simulink model "OrbiterPhysicalSystem"  (R2022b)
settings: Solver=VariableStepAuto  StartTime=0.0  StopTime=100  RelTol=1e-3
libraries: fl_lib x62, nesl_utility x10
settings Model: Creator=aless  LastModifiedBy=aless

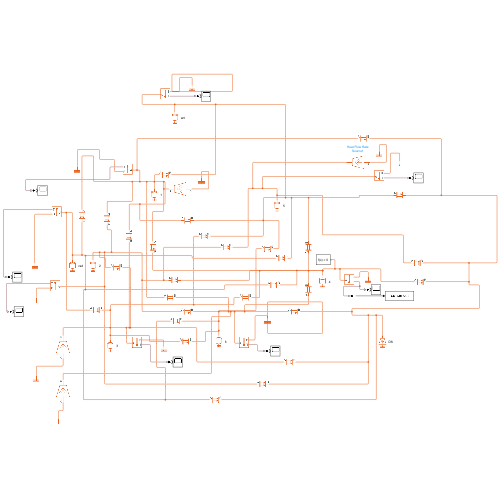
[thumbnail: Simulink's stored preview of the top-level diagram]
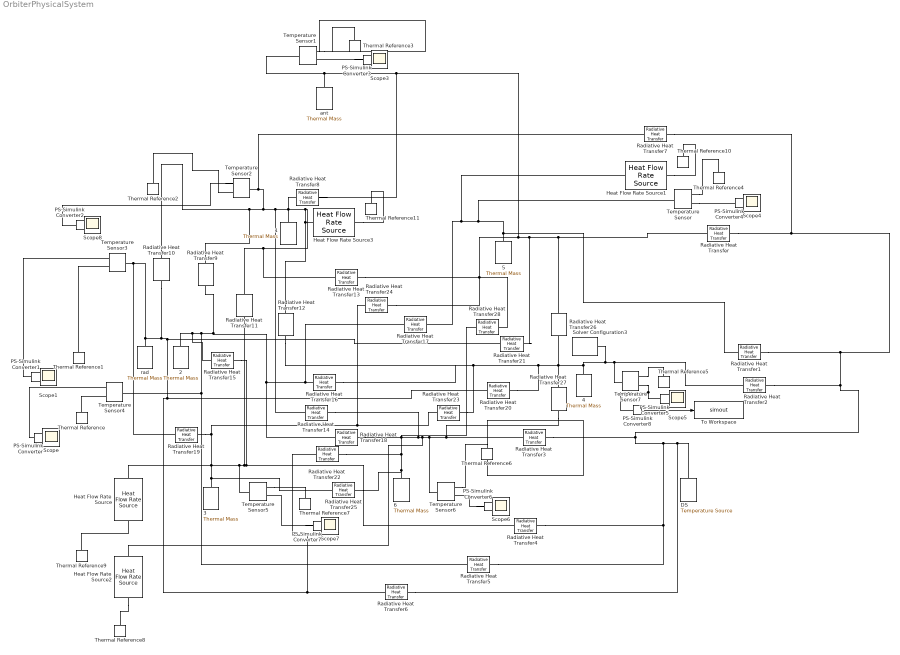
== system OrbiterPhysicalSystem ==
  {1..6} (6 alike) : fl_lib/Thermal/Thermal Elements/Thermal Mass  mass=1 kg  sp_heat=447 J/(K*kg)  num_ports=foundation.enum.numPorts2.one  T_specify=off  T_priority=High  T=300 K  T_nominal_specify=on  T_nominal_unit=K  T_nominal_value=T0  Q_specify=off  Q_priority=None  Q=0 W  Q_nominal_specify=off  Q_nominal_unit=W  Q_nominal_value=1
  DS : fl_lib/Thermal/Thermal Sources/Temperature Source  temperature=4 K
  Heat Flow Rate Source : fl_lib/Thermal/Thermal Sources/Heat Flow Rate Source  heat_flow=Q_ext_hot3 W
      settings: InternalSimscapePortConfiguration="{\"Bottom\":[],\"Left\":[{\"id\":\"B\",\"label\":\"B\",\"type\":\"foundation.thermal.thermal\"}],\"Right\":[{\"id\":\"A\",\"label\":\"A\",\"type\":\"foundation.thermal.thermal\"}],\"Top\":[]}"
  Heat Flow Rate Source1 : fl_lib/Thermal/Thermal Sources/Heat Flow Rate Source  heat_flow=Q_ext_hot5 W
      settings: InternalSimscapePortConfiguration="{\"Bottom\":[],\"Left\":[{\"id\":\"B\",\"label\":\"B\",\"type\":\"foundation.thermal.thermal\"}],\"Right\":[{\"id\":\"A\",\"label\":\"A\",\"type\":\"foundation.thermal.thermal\"}],\"Top\":[]}"
  Heat Flow Rate Source2 : fl_lib/Thermal/Thermal Sources/Heat Flow Rate Source  heat_flow=Q_ext_hot3 W
      settings: InternalSimscapePortConfiguration="{\"Bottom\":[],\"Left\":[{\"id\":\"B\",\"label\":\"B\",\"type\":\"foundation.thermal.thermal\"}],\"Right\":[{\"id\":\"A\",\"label\":\"A\",\"type\":\"foundation.thermal.thermal\"}],\"Top\":[]}"
  Heat Flow Rate Source3 : fl_lib/Thermal/Thermal Sources/Heat Flow Rate Source  heat_flow=Q_hot W
      settings: InternalSimscapePortConfiguration="{\"Bottom\":[],\"Left\":[{\"id\":\"B\",\"label\":\"B\",\"type\":\"foundation.thermal.thermal\"}],\"Right\":[{\"id\":\"A\",\"label\":\"A\",\"type\":\"foundation.thermal.thermal\"}],\"Top\":[]}"
  PS-Simulink Converter{,1..8} (9 alike) : nesl_utility/PS-Simulink Converter  PhysicalDomain=network_engine_domain  SubClassName=ps_output  LeftPortType=input  RightPortType=output  PseudoPeriodic=off  Frequencies=[]  VectorFormat=inherit  Unit=inherit  AffineConversion=off
  Radiative Heat Transfer : fl_lib/Thermal/Thermal Elements/Radiative Heat Transfer  area=A_ant m^2  rad_tr_coeff=R.R_ant0 W/(K^4*m^2)  T_specify=off  T_priority=None  T=0 K  T_nominal_specify=off  T_nominal_unit=K  T_nominal_value=1  Q_specify=off  Q_priority=None  Q=0 W  Q_nominal_specify=off  Q_nominal_unit=W  Q_nominal_value=1
      settings: InternalSimscapePortConfiguration="{\"Bottom\":[],\"Left\":[{\"id\":\"A\",\"label\":\"A\",\"type\":\"foundation.thermal.thermal\"}],\"Right\":[{\"id\":\"B\",\"label\":\"B\",\"type\":\"foundation.thermal.thermal\"}],\"Top\":[]}"
  Radiative Heat Transfer1 : fl_lib/Thermal/Thermal Elements/Radiative Heat Transfer  area=A5 m^2  rad_tr_coeff=R.R_50 W/(K^4*m^2)  T_specify=off  T_priority=None  T=0 K  T_nominal_specify=off  T_nominal_unit=K  T_nominal_value=1  Q_specify=off  Q_priority=None  Q=0 W  Q_nominal_specify=off  Q_nominal_unit=W  Q_nominal_value=1
      settings: InternalSimscapePortConfiguration="{\"Bottom\":[],\"Left\":[{\"id\":\"A\",\"label\":\"A\",\"type\":\"foundation.thermal.thermal\"}],\"Right\":[{\"id\":\"B\",\"label\":\"B\",\"type\":\"foundation.thermal.thermal\"}],\"Top\":[]}"
  Radiative Heat Transfer10 : fl_lib/Thermal/Thermal Elements/Radiative Heat Transfer  area=A1 m^2  rad_tr_coeff=R.R_1rad W/(K^4*m^2)  T_specify=off  T_priority=None  T=0 K  T_nominal_specify=off  T_nominal_unit=K  T_nominal_value=1  Q_specify=off  Q_priority=None  Q=0 W  Q_nominal_specify=off  Q_nominal_unit=W  Q_nominal_value=1
      settings: InternalSimscapePortConfiguration="{\"Bottom\":[],\"Left\":[{\"id\":\"A\",\"label\":\"A\",\"type\":\"foundation.thermal.thermal\"}],\"Right\":[{\"id\":\"B\",\"label\":\"B\",\"type\":\"foundation.thermal.thermal\"}],\"Top\":[]}"
  Radiative Heat Transfer11 : fl_lib/Thermal/Thermal Elements/Radiative Heat Transfer  area=A1 m^2  rad_tr_coeff=R.R_13 W/(K^4*m^2)  T_specify=off  T_priority=None  T=0 K  T_nominal_specify=off  T_nominal_unit=K  T_nominal_value=1  Q_specify=off  Q_priority=None  Q=0 W  Q_nominal_specify=off  Q_nominal_unit=W  Q_nominal_value=1
      settings: InternalSimscapePortConfiguration="{\"Bottom\":[],\"Left\":[{\"id\":\"A\",\"label\":\"A\",\"type\":\"foundation.thermal.thermal\"}],\"Right\":[{\"id\":\"B\",\"label\":\"B\",\"type\":\"foundation.thermal.thermal\"}],\"Top\":[]}"
  Radiative Heat Transfer12 : fl_lib/Thermal/Thermal Elements/Radiative Heat Transfer  area=A1 m^2  rad_tr_coeff=R.R_14 W/(K^4*m^2)  T_specify=off  T_priority=None  T=0 K  T_nominal_specify=off  T_nominal_unit=K  T_nominal_value=1  Q_specify=off  Q_priority=None  Q=0 W  Q_nominal_specify=off  Q_nominal_unit=W  Q_nominal_value=1
      settings: InternalSimscapePortConfiguration="{\"Bottom\":[],\"Left\":[{\"id\":\"A\",\"label\":\"A\",\"type\":\"foundation.thermal.thermal\"}],\"Right\":[{\"id\":\"B\",\"label\":\"B\",\"type\":\"foundation.thermal.thermal\"}],\"Top\":[]}"
  Radiative Heat Transfer13 : fl_lib/Thermal/Thermal Elements/Radiative Heat Transfer  area=A1 m^2  rad_tr_coeff=R.R_15 W/(K^4*m^2)  T_specify=off  T_priority=None  T=0 K  T_nominal_specify=off  T_nominal_unit=K  T_nominal_value=1  Q_specify=off  Q_priority=None  Q=0 W  Q_nominal_specify=off  Q_nominal_unit=W  Q_nominal_value=1
      settings: InternalSimscapePortConfiguration="{\"Bottom\":[],\"Left\":[{\"id\":\"A\",\"label\":\"A\",\"type\":\"foundation.thermal.thermal\"}],\"Right\":[{\"id\":\"B\",\"label\":\"B\",\"type\":\"foundation.thermal.thermal\"}],\"Top\":[]}"
  Radiative Heat Transfer14 : fl_lib/Thermal/Thermal Elements/Radiative Heat Transfer  area=A1 m^2  rad_tr_coeff=R.R_16 W/(K^4*m^2)  T_specify=off  T_priority=None  T=0 K  T_nominal_specify=off  T_nominal_unit=K  T_nominal_value=1  Q_specify=off  Q_priority=None  Q=0 W  Q_nominal_specify=off  Q_nominal_unit=W  Q_nominal_value=1
      settings: InternalSimscapePortConfiguration="{\"Bottom\":[],\"Left\":[{\"id\":\"A\",\"label\":\"A\",\"type\":\"foundation.thermal.thermal\"}],\"Right\":[{\"id\":\"B\",\"label\":\"B\",\"type\":\"foundation.thermal.thermal\"}],\"Top\":[]}"
  Radiative Heat Transfer15 : fl_lib/Thermal/Thermal Elements/Radiative Heat Transfer  area=A2 m^2  rad_tr_coeff=R.R_23 W/(K^4*m^2)  T_specify=off  T_priority=None  T=0 K  T_nominal_specify=off  T_nominal_unit=K  T_nominal_value=1  Q_specify=off  Q_priority=None  Q=0 W  Q_nominal_specify=off  Q_nominal_unit=W  Q_nominal_value=1
      settings: InternalSimscapePortConfiguration="{\"Bottom\":[],\"Left\":[{\"id\":\"A\",\"label\":\"A\",\"type\":\"foundation.thermal.thermal\"}],\"Right\":[{\"id\":\"B\",\"label\":\"B\",\"type\":\"foundation.thermal.thermal\"}],\"Top\":[]}"
  Radiative Heat Transfer16 : fl_lib/Thermal/Thermal Elements/Radiative Heat Transfer  area=A2 m^2  rad_tr_coeff=R.R_24 W/(K^4*m^2)  T_specify=off  T_priority=None  T=0 K  T_nominal_specify=off  T_nominal_unit=K  T_nominal_value=1  Q_specify=off  Q_priority=None  Q=0 W  Q_nominal_specify=off  Q_nominal_unit=W  Q_nominal_value=1
      settings: InternalSimscapePortConfiguration="{\"Bottom\":[],\"Left\":[{\"id\":\"A\",\"label\":\"A\",\"type\":\"foundation.thermal.thermal\"}],\"Right\":[{\"id\":\"B\",\"label\":\"B\",\"type\":\"foundation.thermal.thermal\"}],\"Top\":[]}"
  Radiative Heat Transfer17 : fl_lib/Thermal/Thermal Elements/Radiative Heat Transfer  area=A2 m^2  rad_tr_coeff=R.R_25 W/(K^4*m^2)  T_specify=off  T_priority=None  T=0 K  T_nominal_specify=off  T_nominal_unit=K  T_nominal_value=1  Q_specify=off  Q_priority=None  Q=0 W  Q_nominal_specify=off  Q_nominal_unit=W  Q_nominal_value=1
      settings: InternalSimscapePortConfiguration="{\"Bottom\":[],\"Left\":[{\"id\":\"A\",\"label\":\"A\",\"type\":\"foundation.thermal.thermal\"}],\"Right\":[{\"id\":\"B\",\"label\":\"B\",\"type\":\"foundation.thermal.thermal\"}],\"Top\":[]}"
  Radiative Heat Transfer18 : fl_lib/Thermal/Thermal Elements/Radiative Heat Transfer  area=A2 m^2  rad_tr_coeff=R.R_26 W/(K^4*m^2)  T_specify=off  T_priority=None  T=0 K  T_nominal_specify=off  T_nominal_unit=K  T_nominal_value=1  Q_specify=off  Q_priority=None  Q=0 W  Q_nominal_specify=off  Q_nominal_unit=W  Q_nominal_value=1
      settings: InternalSimscapePortConfiguration="{\"Bottom\":[],\"Left\":[{\"id\":\"A\",\"label\":\"A\",\"type\":\"foundation.thermal.thermal\"}],\"Right\":[{\"id\":\"B\",\"label\":\"B\",\"type\":\"foundation.thermal.thermal\"}],\"Top\":[]}"
  Radiative Heat Transfer19 : fl_lib/Thermal/Thermal Elements/Radiative Heat Transfer  area=A_rad_tot m^2  rad_tr_coeff=R.R_rad3 W/(K^4*m^2)  T_specify=off  T_priority=None  T=0 K  T_nominal_specify=off  T_nominal_unit=K  T_nominal_value=1  Q_specify=off  Q_priority=None  Q=0 W  Q_nominal_specify=off  Q_nominal_unit=W  Q_nominal_value=1
      settings: InternalSimscapePortConfiguration="{\"Bottom\":[],\"Left\":[{\"id\":\"A\",\"label\":\"A\",\"type\":\"foundation.thermal.thermal\"}],\"Right\":[{\"id\":\"B\",\"label\":\"B\",\"type\":\"foundation.thermal.thermal\"}],\"Top\":[]}"
  Radiative Heat Transfer2 : fl_lib/Thermal/Thermal Elements/Radiative Heat Transfer  area=A4 m^2  rad_tr_coeff=R.R_40 W/(K^4*m^2)  T_specify=off  T_priority=None  T=0 K  T_nominal_specify=off  T_nominal_unit=K  T_nominal_value=1  Q_specify=off  Q_priority=None  Q=0 W  Q_nominal_specify=off  Q_nominal_unit=W  Q_nominal_value=1
      settings: InternalSimscapePortConfiguration="{\"Bottom\":[],\"Left\":[{\"id\":\"A\",\"label\":\"A\",\"type\":\"foundation.thermal.thermal\"}],\"Right\":[{\"id\":\"B\",\"label\":\"B\",\"type\":\"foundation.thermal.thermal\"}],\"Top\":[]}"
  Radiative Heat Transfer20 : fl_lib/Thermal/Thermal Elements/Radiative Heat Transfer  area=A_rad_tot m^2  rad_tr_coeff=R.R_rad4 W/(K^4*m^2)  T_specify=off  T_priority=None  T=0 K  T_nominal_specify=off  T_nominal_unit=K  T_nominal_value=1  Q_specify=off  Q_priority=None  Q=0 W  Q_nominal_specify=off  Q_nominal_unit=W  Q_nominal_value=1
      settings: InternalSimscapePortConfiguration="{\"Bottom\":[],\"Left\":[{\"id\":\"A\",\"label\":\"A\",\"type\":\"foundation.thermal.thermal\"}],\"Right\":[{\"id\":\"B\",\"label\":\"B\",\"type\":\"foundation.thermal.thermal\"}],\"Top\":[]}"
  Radiative Heat Transfer21 : fl_lib/Thermal/Thermal Elements/Radiative Heat Transfer  area=A_rad_tot m^2  rad_tr_coeff=R.R_rad5 W/(K^4*m^2)  T_specify=off  T_priority=None  T=0 K  T_nominal_specify=off  T_nominal_unit=K  T_nominal_value=1  Q_specify=off  Q_priority=None  Q=0 W  Q_nominal_specify=off  Q_nominal_unit=W  Q_nominal_value=1
      settings: InternalSimscapePortConfiguration="{\"Bottom\":[],\"Left\":[{\"id\":\"A\",\"label\":\"A\",\"type\":\"foundation.thermal.thermal\"}],\"Right\":[{\"id\":\"B\",\"label\":\"B\",\"type\":\"foundation.thermal.thermal\"}],\"Top\":[]}"
  Radiative Heat Transfer22 : fl_lib/Thermal/Thermal Elements/Radiative Heat Transfer  area=A_rad_tot m^2  rad_tr_coeff=R.R_rad6 W/(K^4*m^2)  T_specify=off  T_priority=None  T=0 K  T_nominal_specify=off  T_nominal_unit=K  T_nominal_value=1  Q_specify=off  Q_priority=None  Q=0 W  Q_nominal_specify=off  Q_nominal_unit=W  Q_nominal_value=1
      settings: InternalSimscapePortConfiguration="{\"Bottom\":[],\"Left\":[{\"id\":\"A\",\"label\":\"A\",\"type\":\"foundation.thermal.thermal\"}],\"Right\":[{\"id\":\"B\",\"label\":\"B\",\"type\":\"foundation.thermal.thermal\"}],\"Top\":[]}"
  Radiative Heat Transfer23 : fl_lib/Thermal/Thermal Elements/Radiative Heat Transfer  area=A3 m^2  rad_tr_coeff=R.R_34 W/(K^4*m^2)  T_specify=off  T_priority=None  T=0 K  T_nominal_specify=off  T_nominal_unit=K  T_nominal_value=1  Q_specify=off  Q_priority=None  Q=0 W  Q_nominal_specify=off  Q_nominal_unit=W  Q_nominal_value=1
      settings: InternalSimscapePortConfiguration="{\"Bottom\":[],\"Left\":[{\"id\":\"A\",\"label\":\"A\",\"type\":\"foundation.thermal.thermal\"}],\"Right\":[{\"id\":\"B\",\"label\":\"B\",\"type\":\"foundation.thermal.thermal\"}],\"Top\":[]}"
  Radiative Heat Transfer24 : fl_lib/Thermal/Thermal Elements/Radiative Heat Transfer  area=A3 m^2  rad_tr_coeff=R.R_35 W/(K^4*m^2)  T_specify=off  T_priority=None  T=0 K  T_nominal_specify=off  T_nominal_unit=K  T_nominal_value=1  Q_specify=off  Q_priority=None  Q=0 W  Q_nominal_specify=off  Q_nominal_unit=W  Q_nominal_value=1
      settings: InternalSimscapePortConfiguration="{\"Bottom\":[],\"Left\":[{\"id\":\"A\",\"label\":\"A\",\"type\":\"foundation.thermal.thermal\"}],\"Right\":[{\"id\":\"B\",\"label\":\"B\",\"type\":\"foundation.thermal.thermal\"}],\"Top\":[]}"
  Radiative Heat Transfer25 : fl_lib/Thermal/Thermal Elements/Radiative Heat Transfer  area=A3 m^2  rad_tr_coeff=R.R_36 W/(K^4*m^2)  T_specify=off  T_priority=None  T=0 K  T_nominal_specify=off  T_nominal_unit=K  T_nominal_value=1  Q_specify=off  Q_priority=None  Q=0 W  Q_nominal_specify=off  Q_nominal_unit=W  Q_nominal_value=1
      settings: InternalSimscapePortConfiguration="{\"Bottom\":[],\"Left\":[{\"id\":\"A\",\"label\":\"A\",\"type\":\"foundation.thermal.thermal\"}],\"Right\":[{\"id\":\"B\",\"label\":\"B\",\"type\":\"foundation.thermal.thermal\"}],\"Top\":[]}"
  Radiative Heat Transfer26 : fl_lib/Thermal/Thermal Elements/Radiative Heat Transfer  area=A4 m^2  rad_tr_coeff=R.R_45 W/(K^4*m^2)  T_specify=off  T_priority=None  T=0 K  T_nominal_specify=off  T_nominal_unit=K  T_nominal_value=1  Q_specify=off  Q_priority=None  Q=0 W  Q_nominal_specify=off  Q_nominal_unit=W  Q_nominal_value=1
      settings: InternalSimscapePortConfiguration="{\"Bottom\":[],\"Left\":[{\"id\":\"A\",\"label\":\"A\",\"type\":\"foundation.thermal.thermal\"}],\"Right\":[{\"id\":\"B\",\"label\":\"B\",\"type\":\"foundation.thermal.thermal\"}],\"Top\":[]}"
  Radiative Heat Transfer27 : fl_lib/Thermal/Thermal Elements/Radiative Heat Transfer  area=A4 m^2  rad_tr_coeff=R.R_46 W/(K^4*m^2)  T_specify=off  T_priority=None  T=0 K  T_nominal_specify=off  T_nominal_unit=K  T_nominal_value=1  Q_specify=off  Q_priority=None  Q=0 W  Q_nominal_specify=off  Q_nominal_unit=W  Q_nominal_value=1
      settings: InternalSimscapePortConfiguration="{\"Bottom\":[],\"Left\":[{\"id\":\"A\",\"label\":\"A\",\"type\":\"foundation.thermal.thermal\"}],\"Right\":[{\"id\":\"B\",\"label\":\"B\",\"type\":\"foundation.thermal.thermal\"}],\"Top\":[]}"
  Radiative Heat Transfer28 : fl_lib/Thermal/Thermal Elements/Radiative Heat Transfer  area=A5 m^2  rad_tr_coeff=R.R_56 W/(K^4*m^2)  T_specify=off  T_priority=None  T=0 K  T_nominal_specify=off  T_nominal_unit=K  T_nominal_value=1  Q_specify=off  Q_priority=None  Q=0 W  Q_nominal_specify=off  Q_nominal_unit=W  Q_nominal_value=1
      settings: InternalSimscapePortConfiguration="{\"Bottom\":[],\"Left\":[{\"id\":\"A\",\"label\":\"A\",\"type\":\"foundation.thermal.thermal\"}],\"Right\":[{\"id\":\"B\",\"label\":\"B\",\"type\":\"foundation.thermal.thermal\"}],\"Top\":[]}"
  Radiative Heat Transfer3 : fl_lib/Thermal/Thermal Elements/Radiative Heat Transfer  area=A6 m^2  rad_tr_coeff=R.R_60 W/(K^4*m^2)  T_specify=off  T_priority=None  T=0 K  T_nominal_specify=off  T_nominal_unit=K  T_nominal_value=1  Q_specify=off  Q_priority=None  Q=0 W  Q_nominal_specify=off  Q_nominal_unit=W  Q_nominal_value=1
      settings: InternalSimscapePortConfiguration="{\"Bottom\":[],\"Left\":[{\"id\":\"A\",\"label\":\"A\",\"type\":\"foundation.thermal.thermal\"}],\"Right\":[{\"id\":\"B\",\"label\":\"B\",\"type\":\"foundation.thermal.thermal\"}],\"Top\":[]}"
  Radiative Heat Transfer4 : fl_lib/Thermal/Thermal Elements/Radiative Heat Transfer  area=A3 m^2  rad_tr_coeff=R.R_30 W/(K^4*m^2)  T_specify=off  T_priority=None  T=0 K  T_nominal_specify=off  T_nominal_unit=K  T_nominal_value=1  Q_specify=off  Q_priority=None  Q=0 W  Q_nominal_specify=off  Q_nominal_unit=W  Q_nominal_value=1
      settings: InternalSimscapePortConfiguration="{\"Bottom\":[],\"Left\":[{\"id\":\"A\",\"label\":\"A\",\"type\":\"foundation.thermal.thermal\"}],\"Right\":[{\"id\":\"B\",\"label\":\"B\",\"type\":\"foundation.thermal.thermal\"}],\"Top\":[]}"
  Radiative Heat Transfer5 : fl_lib/Thermal/Thermal Elements/Radiative Heat Transfer  area=A2 m^2  rad_tr_coeff=R.R_20 W/(K^4*m^2)  T_specify=off  T_priority=None  T=0 K  T_nominal_specify=off  T_nominal_unit=K  T_nominal_value=1  Q_specify=off  Q_priority=None  Q=0 W  Q_nominal_specify=off  Q_nominal_unit=W  Q_nominal_value=1
      settings: InternalSimscapePortConfiguration="{\"Bottom\":[],\"Left\":[{\"id\":\"A\",\"label\":\"A\",\"type\":\"foundation.thermal.thermal\"}],\"Right\":[{\"id\":\"B\",\"label\":\"B\",\"type\":\"foundation.thermal.thermal\"}],\"Top\":[]}"
  Radiative Heat Transfer6 : fl_lib/Thermal/Thermal Elements/Radiative Heat Transfer  area=A_rad_tot m^2  rad_tr_coeff=R.R_rad0 W/(K^4*m^2)  T_specify=off  T_priority=None  T=0 K  T_nominal_specify=off  T_nominal_unit=K  T_nominal_value=1  Q_specify=off  Q_priority=None  Q=0 W  Q_nominal_specify=off  Q_nominal_unit=W  Q_nominal_value=1
      settings: InternalSimscapePortConfiguration="{\"Bottom\":[],\"Left\":[{\"id\":\"A\",\"label\":\"A\",\"type\":\"foundation.thermal.thermal\"}],\"Right\":[{\"id\":\"B\",\"label\":\"B\",\"type\":\"foundation.thermal.thermal\"}],\"Top\":[]}"
  Radiative Heat Transfer7 : fl_lib/Thermal/Thermal Elements/Radiative Heat Transfer  area=A1 m^2  rad_tr_coeff=R.R_10 W/(K^4*m^2)  T_specify=off  T_priority=None  T=0 K  T_nominal_specify=off  T_nominal_unit=K  T_nominal_value=1  Q_specify=off  Q_priority=None  Q=0 W  Q_nominal_specify=off  Q_nominal_unit=W  Q_nominal_value=1
      settings: InternalSimscapePortConfiguration="{\"Bottom\":[],\"Left\":[{\"id\":\"A\",\"label\":\"A\",\"type\":\"foundation.thermal.thermal\"}],\"Right\":[{\"id\":\"B\",\"label\":\"B\",\"type\":\"foundation.thermal.thermal\"}],\"Top\":[]}"
  Radiative Heat Transfer8 : fl_lib/Thermal/Thermal Elements/Radiative Heat Transfer  area=A1 m^2  rad_tr_coeff=R.R_1ant W/(K^4*m^2)  T_specify=off  T_priority=None  T=0 K  T_nominal_specify=off  T_nominal_unit=K  T_nominal_value=1  Q_specify=off  Q_priority=None  Q=0 W  Q_nominal_specify=off  Q_nominal_unit=W  Q_nominal_value=1
      settings: InternalSimscapePortConfiguration="{\"Bottom\":[],\"Left\":[{\"id\":\"A\",\"label\":\"A\",\"type\":\"foundation.thermal.thermal\"}],\"Right\":[{\"id\":\"B\",\"label\":\"B\",\"type\":\"foundation.thermal.thermal\"}],\"Top\":[]}"
  Radiative Heat Transfer9 : fl_lib/Thermal/Thermal Elements/Radiative Heat Transfer  area=A1 m^2  rad_tr_coeff=R.R_12 W/(K^4*m^2)  T_specify=off  T_priority=None  T=0 K  T_nominal_specify=off  T_nominal_unit=K  T_nominal_value=1  Q_specify=off  Q_priority=None  Q=0 W  Q_nominal_specify=off  Q_nominal_unit=W  Q_nominal_value=1
      settings: InternalSimscapePortConfiguration="{\"Bottom\":[],\"Left\":[{\"id\":\"A\",\"label\":\"A\",\"type\":\"foundation.thermal.thermal\"}],\"Right\":[{\"id\":\"B\",\"label\":\"B\",\"type\":\"foundation.thermal.thermal\"}],\"Top\":[]}"
  Scope{,1,3..8} (8 alike) : Scope
  Solver Configuration3 : nesl_utility/Solver Configuration  PhysicalDomain=network_engine_domain  SubClassName=solver  LeftPortType=input  RightPortType=generic  Tones=[]  Harmonics=[]  SimulateNoise=off  Profile=off  UseLocalSampling=off  EnableSwitchedLinearOptims=on  FrequencyDomain=off  UseCCode=off  RelTol=0.001  AbsTol=0.001  MinStep=1e-09  ToWorkspace=off  RevertToSquareIcSolve=off  NumHomotopyIterations=100  PhasorMode=off  PhasorModeNumHarmonics=1  ConsistencySolver=NEWTON_XTOL_AFTER_FTOL  IndexReductionMethod=DerivativeReplacement  DoDC=off  ResidualTolerance=1e-09  ConsistencyTolSource=GLOBAL  ConsistencyAbsTol=0.001  ConsistencyRelTol=0.001  ConsistencyTolFactor=0.001  UseLocalSolver=off  LocalSolverChoice=NE_BACKWARD_EULER_ADVANCER  ResolveIndetEquations=on  FunctionEvalNumThread=1  LocalSolverSampleTime=0.001  DoFixedCost=off  MaxNonlinIter=3  MaxModeIter=2  ComputeImpulses=off  ImpulseIterations=2  LinearAlgebra=auto  LinearAlgebraNumThread=0  EquationFormulation=NE_TIME_EF  DelaysMemoryBudget=1024  AutomaticFiltering=on  FilteringTimeConstant=0.001  PartitionStorageMethod=AS_NEEDED  PartitionMemoryBudget=1024  PartitionMethod=ROBUST
  Temperature Sensor{,1..7} (8 alike) : fl_lib/Thermal/Thermal Sensors/Temperature Sensor
  Thermal Reference{,1..11} (12 alike) : fl_lib/Thermal/Thermal Elements/Thermal Reference
  To Workspace : ToWorkspace  VariableName=simout  SaveFormat=Timeseries  SampleTime=-1
  ant : fl_lib/Thermal/Thermal Elements/Thermal Mass  mass=1 kg  sp_heat=447 J/(K*kg)  num_ports=foundation.enum.numPorts2.one  T_specify=off  T_priority=High  T=300 K  T_nominal_specify=on  T_nominal_unit=K  T_nominal_value=T0  Q_specify=off  Q_priority=None  Q=0 W  Q_nominal_specify=off  Q_nominal_unit=W  Q_nominal_value=1
  rad : fl_lib/Thermal/Thermal Elements/Thermal Mass  mass=1 kg  sp_heat=447 J/(K*kg)  num_ports=foundation.enum.numPorts2.one  T_specify=off  T_priority=High  T=300 K  T_nominal_specify=on  T_nominal_unit=K  T_nominal_value=T0  Q_specify=off  Q_priority=None  Q=0 W  Q_nominal_specify=off  Q_nominal_unit=W  Q_nominal_value=1
  wires:
  PS-Simulink Converter8/1 -> To Workspace/1
  connections:
  Radiative Heat Transfer/RConn1 -- Radiative Heat Transfer7/RConn1 -- Radiative Heat Transfer1/RConn1 -- Radiative Heat Transfer2/RConn1 -- Radiative Heat Transfer3/RConn1 -- Radiative Heat Transfer4/RConn1 -- Radiative Heat Transfer5/RConn1 -- Radiative Heat Transfer6/RConn1 -- DS/LConn1
  ant/LConn1 -- Temperature Sensor1/LConn1 -- Radiative Heat Transfer8/RConn1 -- Radiative Heat Transfer28/RConn1 -- Radiative Heat Transfer24/RConn1 -- Radiative Heat Transfer13/RConn1 -- Radiative Heat Transfer21/RConn1 -- Radiative Heat Transfer26/RConn1 -- Radiative Heat Transfer/LConn1
  5/LConn1 -- Heat Flow Rate Source1/LConn1 -- Radiative Heat Transfer17/RConn1 -- Temperature Sensor/LConn1 -- Radiative Heat Transfer1/LConn1
  4/LConn1 -- Radiative Heat Transfer26/LConn1 -- Radiative Heat Transfer27/RConn1 -- Radiative Heat Transfer23/RConn1 -- Radiative Heat Transfer16/RConn1 -- Radiative Heat Transfer20/RConn1 -- Radiative Heat Transfer12/RConn1 -- Solver Configuration3/RConn1 -- Temperature Sensor7/LConn1 -- Radiative Heat Transfer2/LConn1
  6/LConn1 -- Radiative Heat Transfer25/RConn1 -- Radiative Heat Transfer28/LConn1 -- Radiative Heat Transfer18/RConn1 -- Radiative Heat Transfer14/RConn1 -- Heat Flow Rate Source2/LConn1 -- Temperature Sensor6/LConn1 -- Radiative Heat Transfer27/LConn1 -- Radiative Heat Transfer3/LConn1 -- Radiative Heat Transfer22/RConn1
  3/LConn1 -- Radiative Heat Transfer25/LConn1 -- Radiative Heat Transfer24/LConn1 -- Radiative Heat Transfer23/LConn1 -- Radiative Heat Transfer19/RConn1 -- Heat Flow Rate Source/LConn1 -- Radiative Heat Transfer15/RConn1 -- Radiative Heat Transfer4/LConn1 -- Radiative Heat Transfer11/RConn1 -- Temperature Sensor5/LConn1
  2/LConn1 -- Radiative Heat Transfer15/LConn1 -- Radiative Heat Transfer18/LConn1 -- Radiative Heat Transfer17/LConn1 -- Radiative Heat Transfer16/LConn1 -- Radiative Heat Transfer9/RConn1 -- Temperature Sensor4/LConn1 -- Radiative Heat Transfer5/LConn1
  rad/LConn1 -- Radiative Heat Transfer10/RConn1 -- Radiative Heat Transfer20/LConn1 -- Radiative Heat Transfer22/LConn1 -- Radiative Heat Transfer6/LConn1 -- Radiative Heat Transfer21/LConn1 -- Radiative Heat Transfer19/LConn1 -- Temperature Sensor3/LConn1
  1/LConn1 -- Radiative Heat Transfer13/LConn1 -- Radiative Heat Transfer11/LConn1 -- Heat Flow Rate Source3/LConn1 -- Radiative Heat Transfer12/LConn1 -- Radiative Heat Transfer14/LConn1 -- Radiative Heat Transfer10/LConn1 -- Radiative Heat Transfer9/LConn1 -- Radiative Heat Transfer7/LConn1 -- Temperature Sensor2/LConn1 -- Radiative Heat Transfer8/LConn1
  Temperature Sensor4/RConn2 -- PS-Simulink Converter/LConn1
  Thermal Reference/LConn1 -- Temperature Sensor4/RConn1
  Temperature Sensor3/RConn2 -- PS-Simulink Converter1/LConn1
  Thermal Reference1/LConn1 -- Temperature Sensor3/RConn1
  Thermal Reference2/LConn1 -- Temperature Sensor2/RConn1
  PS-Simulink Converter3/LConn1 -- Temperature Sensor1/RConn2
  Temperature Sensor1/RConn1 -- Thermal Reference3/LConn1
  Temperature Sensor/RConn2 -- PS-Simulink Converter4/LConn1
  Temperature Sensor/RConn1 -- Thermal Reference4/LConn1
  Temperature Sensor7/RConn2 -- PS-Simulink Converter8/LConn1 -- PS-Simulink Converter5/LConn1
  Temperature Sensor7/RConn1 -- Thermal Reference5/LConn1
  PS-Simulink Converter6/LConn1 -- Temperature Sensor6/RConn2
  Temperature Sensor6/RConn1 -- Thermal Reference6/LConn1
  PS-Simulink Converter7/LConn1 -- Temperature Sensor5/RConn2
  Temperature Sensor5/RConn1 -- Thermal Reference7/LConn1
  Temperature Sensor2/RConn2 -- PS-Simulink Converter2/LConn1
  Heat Flow Rate Source2/RConn1 -- Thermal Reference8/LConn1
  Thermal Reference9/LConn1 -- Heat Flow Rate Source/RConn1
  Heat Flow Rate Source1/RConn1 -- Thermal Reference10/LConn1
  Heat Flow Rate Source3/RConn1 -- Thermal Reference11/LConn1
